simulink model "fullstate_servo_sim"  (R2020a)
settings: Solver=FixedStepAuto  StartTime=0.0  StopTime=30  FixedStep=0.002  RelTol=1e-6
undefined symbols (not defined in the file): icd, K, Ka, sysd_full, T
libraries: simulink_extras x1
settings Model: Creator=Jasper  LastModifiedBy=Jasper

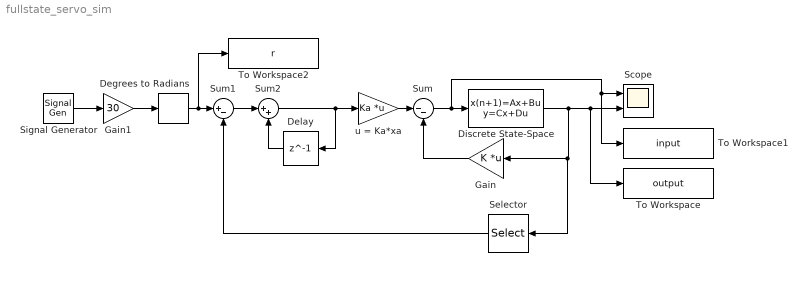
== system fullstate_servo_sim ==
  Degrees to Radians : simulink_extras/Transformations/Degrees to Radians
  Delay : Delay  DelayLength=1  SampleTime=T
  Discrete State-Space : DiscreteStateSpace  A=sysd_full.A  B=sysd_full.B  C=sysd_full.C  D=sysd_full.D  InitialCondition=icd  SampleTime=T
  Gain : Gain  Gain=K  Multiplication=Matrix(K*u)
  Gain1 : Gain  Gain=30
  Scope : Scope  NumInputPorts=2
  Selector : Selector  InputPortWidth=4  IndexOptions=Index vector (dialog)  Indices=[1]  OutputSizes=1
  Signal Generator : SignalGenerator  WaveForm=square  Frequency=0.125
  Sum : Sum  Inputs=|--
  Sum1 : Sum  Inputs=|+-
  Sum2 : Sum  Inputs=|++
  To Workspace : ToWorkspace  VariableName=output  SaveFormat=Timeseries  SampleTime=-1
  To Workspace1 : ToWorkspace  VariableName=input  SaveFormat=Timeseries  SampleTime=-1
  To Workspace2 : ToWorkspace  VariableName=r  SaveFormat=Timeseries  SampleTime=-1
  u = Ka*xa : Gain  Gain=Ka  Multiplication=Matrix(K*u)
  wires:
  Discrete State-Space/1 -> To Workspace/1, Scope/2, Selector/1, Gain/1
  Gain/1 -> Sum/2
  Sum/1 -> Discrete State-Space/1, To Workspace1/1, Scope/1
  Gain1/1 -> Degrees to Radians/1
  Signal Generator/1 -> Gain1/1
  Degrees to Radians/1 -> To Workspace2/1, Sum1/1
  Selector/1 -> Sum1/2
  u = Ka*xa/1 -> Sum/1
  Sum1/1 -> Sum2/1
  Delay/1 -> Sum2/2
  Sum2/1 -> Delay/1, u = Ka*xa/1
